simulink model "nomal_regulator"  (R2019a)
settings: Solver=FixedStepAuto  StartTime=0.0  StopTime=inf  FixedStep=sT  RelTol=1e-3  EnableMultiTasking=on
InitFcn:
  | clear;
  | init_robot;
  | param;
values from neighbouring files (symbols this model uses):
  g = 9.80665    [param.m]    (also in sim_param.m)
  inix = [0.00 0.00]'    [param.m]    (also in sim_param.m)
  iniXzmax = 0.05    [param.m]    (also in sim_param.m)
  iniXzmin = -0.05    [param.m]    (also in sim_param.m)
  iniy = [0.00 0.00]'    [param.m]    (also in sim_param.m)
  iniYzmax = 0.0625    [param.m]    (also in sim_param.m)
  iniYzmin = -0.0625    [param.m]    (also in sim_param.m)
  R = 20    [param.m]    (also in sim_param.m = 1)
  sT = 0.02    [param.m]    (also in sim_param.m = 0.001)
  w = sqrt(g/zc)    [param.m]    (also in sim_param.m)
undefined symbols (not defined in the file or in its folder): Ad, Bd, Cd, Dd, DiscIntNeverNeededParam, Discrete, fdesignblkfcn, gcbh, Time
libraries: raspberrypilib x6, cstblocks x5, dspfdesign x2, ctrlSharedLib x2
settings Model: SimulationMode=external  Creator=hideaki  LastModifiedBy=hideaki
settings SolverCC: PositivePriorityOrder=on
settings OptimizationCC: EnhancedBackFolding=on  PassReuseOutputArgsAs=Individual arguments  MaxStackSize=64  OptimizeBlockOrder=speed  DifferentSizesBufferReuse=on  OptimizationCustomize=off
settings DebuggingCC: ParameterTunabilityLossMsg=error  UnderSpecifiedDimensionMsg=warning
settings HardwareCC: ProdBitPerPointer=32  ProdBitPerSizeT=32  ProdBitPerPtrDiffT=32  ProdLargestAtomicInteger=Long  ProdLargestAtomicFloat=Double  ProdWordSize=32  ProdLongLongMode=on  ProdHWDeviceType=ARM Compatible->ARM Cortex  UseEmbeddedCoderFeatures=off  UseSimulinkCoderFeatures=off
settings SFSimCC: MATLABDynamicMemAlloc=off
settings RTWCC: SystemTargetFile=ert.tlc  HardwareBoard=Raspberry Pi  TLCOptions="-aInlineSetEventsForThisBaseRateFcn=TLC_FALSE -aSuppressMultiTaskScheduler=TLC_FALSE  -aRateBasedStepFcn=0"  TemplateMakefile=ert_default_tmf  RTWVerbose=off  Toolchain=GNU GCC Raspberry Pi  BuildConfiguration=Faster Runs  IncludeHyperlinkInReport=on
settings CodeAppCC: ForceParamTrailComments=on  OperatorAnnotations=on  SimulinkDataObjDesc=on  SFDataObjDesc=on  MangleLength=10  InsertBlockDesc=on
settings ERTTargetCC: SupportNonInlinedSFcns=on  SupportVariableSizeSignals=on  ExtMode=on  ExtModeMexArgs='192.168.10.103' 0 17725  ERTSrcFileBannerTemplate=codertarget_code_template.cgt  ERTHdrFileBannerTemplate=codertarget_code_template.cgt  ERTDataSrcFileTemplate=codertarget_code_template.cgt  ERTDataHdrFileTemplate=codertarget_code_template.cgt

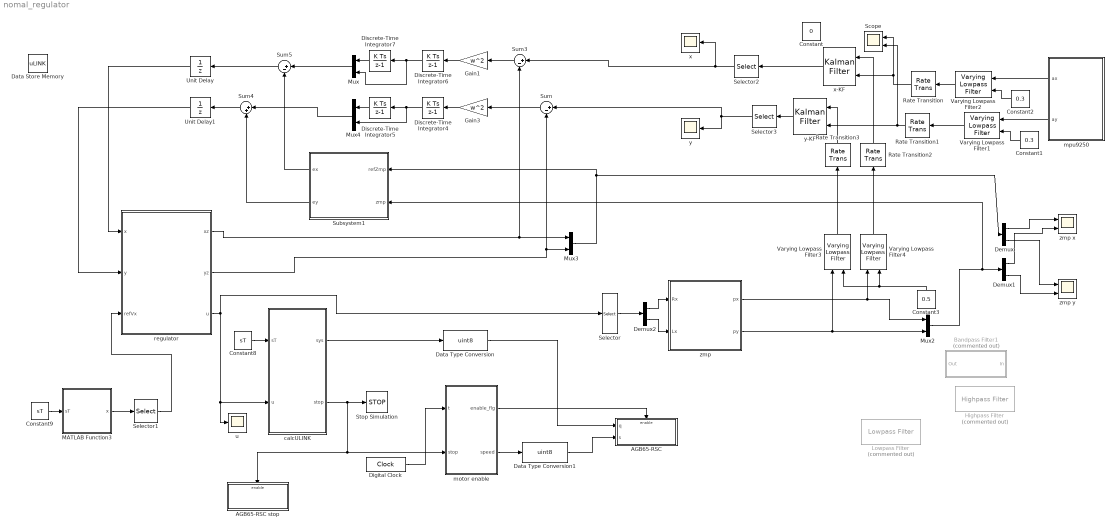
== system nomal_regulator ==
  AGB65-RSC : Subsystem  TreatAsAtomicUnit=on
  AGB65-RSC stop : Subsystem  TreatAsAtomicUnit=on
  Bandpass Filter1 : Subsystem  Commented=on  DialogController=fdesignblkfcn  InitFcn=fdesignblkfcn(gcbh, {'InitFcn'});  mask(Bandpass Filter){}
      mask help: Design a bandpass filter
      settings: CopyFcn=fdesignblkfcn(gcbh, {'CopyFcn'});
      mask Help: helpview(mapfilelocation('dsp'), 'dspbandpassfilter');
      mask Display: disp('Bandpass');
  Constant : Constant  Value=0
  Constant1 : Constant  Value=0.3
  Constant2 : Constant  Value=0.3
  Constant3 : Constant  Value=0.5
  Constant8 : Constant  Value=sT
  Constant9 : Constant  Value=sT
  Data Store Memory : DataStoreMemory  DataStoreName=uLINK  ReadBeforeWriteMsg=warning  WriteAfterWriteMsg=warning  WriteAfterReadMsg=warning  InitialValue=uLINK  ShowAdditionalParam=off  OutDataTypeStr=Bus: ULINK  Dimensions=[15 1]
  Data Type Conversion : DataTypeConversion  OutDataTypeStr=uint8
  Data Type Conversion1 : DataTypeConversion  OutDataTypeStr=uint8
  Demux : Demux  Outputs=2
  Demux1 : Demux  Outputs=2
  Demux2 : Demux  Outputs=2
  Digital Clock : DigitalClock  SampleTime=sT
  Discrete-Time Integrator{4..7} (4 alike) : DiscreteIntegrator  gainval=1  SampleTime=-1  ICPrevOutput=DiscIntNeverNeededParam  ICPrevScaledInput=DiscIntNeverNeededParam
  Gain1 : Gain  Gain=w^2
  Gain3 : Gain  Gain=w^2
  Highpass Filter : dspfdesign/Highpass Filter  Commented=on  FilterType=FIR  DesignForMinimumOrder=on  FilterOrder=50  StopbandFrequency=8e3  PassbandFrequency=12e3  StopbandAttenuation=80  PassbandRipple=0.1  InheritSampleRate=off  SampleRate=44100  SimulateUsing=Interpreted execution  roundingMode=Floor  coeffsDataTypeStr=fixdt(1,16)
      settings: SourceProductName=DSP System Toolbox
  Lowpass Filter : dspfdesign/Lowpass Filter  Commented=on  FilterType=FIR  DesignForMinimumOrder=on  FilterOrder=50  PassbandFrequency=8e3  StopbandFrequency=12e3  PassbandRipple=0.1  StopbandAttenuation=80  InheritSampleRate=off  SampleRate=44100  SimulateUsing=Interpreted execution  roundingMode=Floor  coeffsDataTypeStr=fixdt(1,16)
  MATLAB Function3 : MATLAB Function  TreatAsAtomicUnit=on  SystemSampleTime=sT
  Mux{,2..4} (4 alike) : Mux  Inputs=2
  Rate Transition{,1..3} (4 alike) : RateTransition
  Scope : Scope  NumInputPorts=2
  Selector : Selector  InputPortWidth=8  IndexOptions=Index vector (dialog)  Indices=[3 6]  OutputSizes=1
  Selector1 : Selector  InputPortWidth=3  IndexOptions=Index vector (dialog)  Indices=[2]  OutputSizes=1
  Selector2 : Selector  InputPortWidth=2  IndexOptions=Index vector (dialog)  Indices=[1]  OutputSizes=1
  Selector3 : Selector  InputPortWidth=2  IndexOptions=Index vector (dialog)  Indices=[1]  OutputSizes=1
  Stop Simulation : Stop
  Subsystem1 : Subsystem
  Sum : Sum  Inputs=|+-
  Sum3 : Sum  Inputs=|+-
  Sum4 : Sum  Inputs=|++
  Sum5 : Sum  Inputs=|+-
  Unit Delay : UnitDelay  SampleTime=-1  HasFrameUpgradeWarning=on
  Unit Delay1 : UnitDelay  SampleTime=-1  HasFrameUpgradeWarning=on
  Varying Lowpass Filter{1..4} (4 alike) : cstblocks/Linear Parameter Varying/Varying Lowpass Filter  N=1
      settings: SourceProductName=Control System Toolbox
  calcULINK : MATLAB Function  TreatAsAtomicUnit=on
  motor enable : MATLAB Function  TreatAsAtomicUnit=on
  mpu9250 : Subsystem
  regulator : Subsystem
  u : Scope
  x : Scope
  x-KF : ctrlSharedLib/Kalman Filter  TimeDomain=Discrete-Time  UseCurrentEstimator=on  ModelSource=Individual A, B, C, D matrices  ModelSourceVariable=ss(0.95,1,1,0,1)  A=Ad  B=Bd  C=Cd  D=Dd  NumberOfStates=1  NumberOfInputs=1  NumberOfOutputs=1  InitialEstimateSource=Dialog  X0=inix  P0=[100 50]'  UseK=off  UseGH=off  NumberOfProcessNoiseInputs=1  G=[0 0]'  TimeInvariantG=on  H=10  TimeInvariantH=on  Q=Q  TimeInvariantQ=on  R=R  TimeInvariantR=on  N=0  TimeInvariantN=on  AddInputPort=on  AddEnablePort=off  OutputEstimatedY=off  OutputP=off  Ts=sT
      settings: SourceProductBaseCode=CT
  y : Scope
  y-KF : ctrlSharedLib/Kalman Filter  TimeDomain=Discrete-Time  UseCurrentEstimator=on  ModelSource=Individual A, B, C, D matrices  ModelSourceVariable=ss(0.95,1,1,0,1)  A=Ad  B=Bd  C=Cd  D=Dd  NumberOfStates=1  NumberOfInputs=1  NumberOfOutputs=1  InitialEstimateSource=Dialog  X0=iniy  P0=10  UseK=off  UseGH=off  NumberOfProcessNoiseInputs=1  G=[0 0]'  TimeInvariantG=on  H=10  TimeInvariantH=on  Q=Q  TimeInvariantQ=on  R=R  TimeInvariantR=on  N=0  TimeInvariantN=on  AddInputPort=on  AddEnablePort=off  OutputEstimatedY=off  OutputP=off  Ts=sT
      settings: SourceProductBaseCode=CT
  zmp : Subsystem
  zmp x : Scope  NumInputPorts=2
  zmp y : Scope  NumInputPorts=2
  wires:
  Constant8/1 -> calcULINK/1(sT)
  Constant9/1 -> MATLAB Function3/1(sT)
  mpu9250/1(ax) -> Varying Lowpass Filter2/1
  Digital Clock/1 -> motor enable/1(t)
  Data Type Conversion1/1 -> AGB65-RSC/2(s)
  motor enable/1(enable_flg) -> AGB65-RSC/Enable
  Data Type Conversion/1 -> AGB65-RSC/1(q)
  calcULINK/1(sys) -> Data Type Conversion/1
  motor enable/2(speed) -> Data Type Conversion1/1
  calcULINK/2(stop) -> AGB65-RSC stop/Enable, motor enable/2(stop), Stop Simulation/1
  regulator/3(u) -> u/1, calcULINK/2(u), Selector/1
  Mux2/1 -> Subsystem1/2(zmp), Demux1/1
  Selector/1 -> Demux2/1
  Sum5/1 -> Unit Delay/1
  Sum4/1 -> Unit Delay1/1
  Mux3/1 -> Demux/1, Subsystem1/1(refZmp)
  MATLAB Function3/1(x) -> Selector1/1
  Selector1/1 -> regulator/3(refVx)
  zmp/1(px) -> Varying Lowpass Filter4/1, Mux2/1
  zmp/2(py) -> Mux2/2, Varying Lowpass Filter3/1
  Demux2/1 -> zmp/1(Rx)
  Demux2/2 -> zmp/2(Lx)
  Varying Lowpass Filter2/1 -> Rate Transition/1
  Selector2/1 -> x/1, Sum3/1
  regulator/1(xz) -> Mux3/1, Sum3/2
  regulator/2(yz) -> Mux3/2, Sum/2
  Mux/1 -> Sum5/1
  Demux/1 -> zmp x/1
  Demux1/1 -> zmp x/2
  Demux/2 -> zmp y/1
  Demux1/2 -> zmp y/2
  Discrete-Time Integrator5/1 -> Mux4/1
  Discrete-Time Integrator4/1 -> Discrete-Time Integrator5/1, Mux4/2
  Gain3/1 -> Discrete-Time Integrator4/1
  Sum/1 -> Gain3/1
  Mux4/1 -> Sum4/1
  Selector3/1 -> Sum/1, y/1
  mpu9250/2(ay) -> Varying Lowpass Filter1/1
  Varying Lowpass Filter1/1 -> Rate Transition1/1
  Sum3/1 -> Gain1/1
  Discrete-Time Integrator7/1 -> Mux/1
  Gain1/1 -> Discrete-Time Integrator6/1
  Discrete-Time Integrator6/1 -> Mux/2, Discrete-Time Integrator7/1
  x-KF/1 -> Selector2/1
  y-KF/1 -> Selector3/1
  Constant1/1 -> Varying Lowpass Filter1/2
  Rate Transition/1 -> Scope/1, x-KF/2
  Rate Transition1/1 -> Scope/2, y-KF/2
  Constant2/1 -> Varying Lowpass Filter2/2
  Unit Delay/1 -> regulator/1(x)
  Unit Delay1/1 -> regulator/2(y)
  Subsystem1/1(ex) -> Sum5/2
  Subsystem1/2(ey) -> Sum4/2
  Constant3/1 -> Varying Lowpass Filter3/2, Varying Lowpass Filter4/2
  Varying Lowpass Filter3/1 -> Rate Transition3/1
  Varying Lowpass Filter4/1 -> Rate Transition2/1
  Rate Transition2/1 -> x-KF/1
  Rate Transition3/1 -> y-KF/1

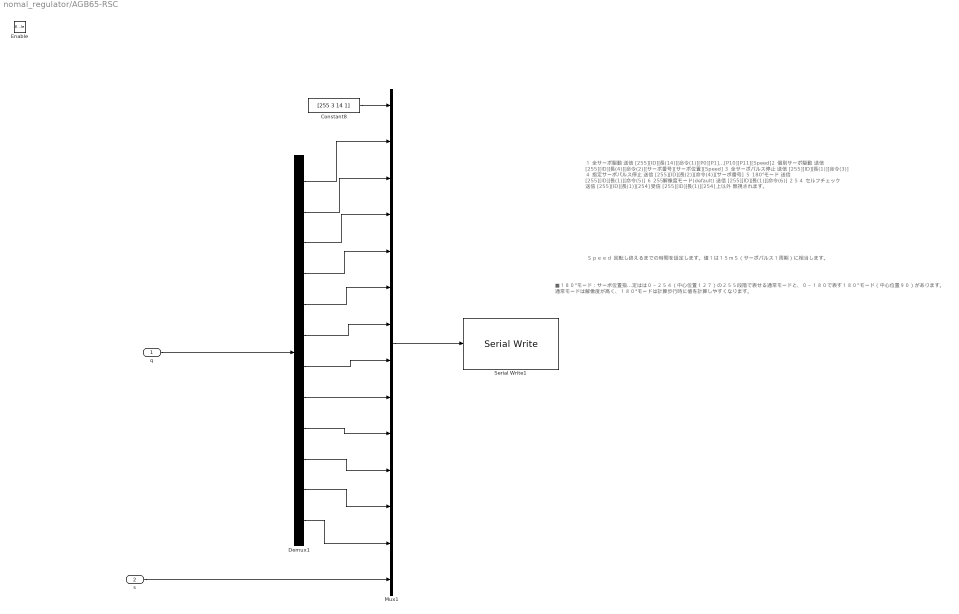
== system nomal_regulator/AGB65-RSC ==
  note: Ｓｐｅｅｄ 回転し終えるまでの時間を設定します。値１は１５ｍＳ（サーボパルス１周期）に相当します。
  note: １ 全サーボ駆動 送信 [255][ID][長(14)][命令(1)][P0][P1]...[P10][P11][Speed]
      | ２ 個別サーボ駆動 送信 [255][ID][長(4)][命令(2)][サーボ番号][サーボ位置][Speed]
      | ３ 全サーボパルス停止 送信 [255][ID][長(1)][命令(3)]
      | ４ 指定サーボパルス停止 送信 [255][ID][長(2)][命令(4)][サーボ番号]
      | ５ 180°モード 送信 [255][ID][長(1)][命令(5)]
      | ６ 255解像度モード(default) 送信 [255][ID][長(1)][命令(6)]
      | ２５４ セルフチェック 送信 [255][ID][長(1)][254] 受信 [255][ID][長(1)][254]
      | 上以外 無視されます。
  note: ■１８０°モード：サーボ位置指定はは０～２５４（中心位置１２７）の２５５段階で表せる通常モードと、０～１８０で表す１８０°モード（中心位置９０）があります。
      | 通常モードは解像度が高く、１８０°モードは計算歩行時に値を計算しやすくなります。
  q : Inport
  s : Inport  Port=2
  Enable : EnablePort
  Constant8 : Constant  Value=[255 3 14 1]  OutDataTypeStr=uint8
  Demux1 : Demux  Outputs=12
  Mux1 : Mux  Inputs=14
  Serial Write1 : raspberrypilib/Serial Write  Priority=1  board=Pi 3 Model B  SCIModule_=/dev/ttyS0  Baudrate_=115200  Parity=None  StopBits_=1  HardwareFlowControl=None  ByteOrder=LittleEndian  OutputStatus=off  blockPlatform=RaspberryPi
      settings: SourceProductName=Simulink Support Package for Raspberry Pi Hardware  SourceProductBaseCode=RASPPI
  wires:
  Constant8/1 -> Mux1/1
  Demux1/11 -> Mux1/12
  q/1 -> Demux1/1
  Demux1/1 -> Mux1/2
  Demux1/3 -> Mux1/4
  Demux1/2 -> Mux1/3
  Mux1/1 -> Serial Write1/1
  Demux1/6 -> Mux1/7
  Demux1/10 -> Mux1/11
  Demux1/5 -> Mux1/6
  Demux1/7 -> Mux1/8
  Demux1/8 -> Mux1/9
  s/1 -> Mux1/14
  Demux1/9 -> Mux1/10
  Demux1/12 -> Mux1/13
  Demux1/4 -> Mux1/5

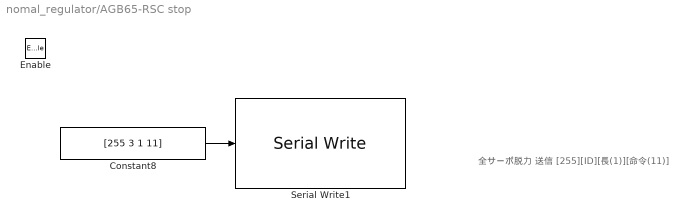
== system nomal_regulator/AGB65-RSC stop ==
  note: 全サーボ脱力 送信 [255][ID][長(1)][命令(11)]
  Enable : EnablePort
  Constant8 : Constant  Value=[255 3 1 11]  OutDataTypeStr=uint8
  Serial Write1 : raspberrypilib/Serial Write  Priority=1  board=Pi 3 Model B  SCIModule_=/dev/ttyS0  Baudrate_=115200  Parity=None  StopBits_=1  HardwareFlowControl=None  ByteOrder=LittleEndian  OutputStatus=off  blockPlatform=RaspberryPi
      settings: SourceProductName=Simulink Support Package for Raspberry Pi Hardware  SourceProductBaseCode=RASPPI
  wires:
  Constant8/1 -> Serial Write1/1

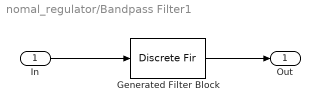
== system nomal_regulator/Bandpass Filter1 ==
  In : Inport
  Generated Filter Block : DiscreteFir  Tag=BlockMethodSubSystem  Coefficients=[-0.0118199987408042547 0.0121628797113327459 0.0187653420961211015 -0.0038859566916752521 0.00617302703660450782 -0.00799330781446441763 0.000649387236100319384 -0.00853505115886610786 -0.00350492002495765911 -0.00711106285974247646 -0.00734644359199590827 -0.00366446356246431793 -0.0101474907261420427 0.00166119112740601912 -0.0106818164382490588 0.00798118016776340478 -0.00794958057228637403 0.0136739609401164072 -0.0017104366339399206 0.0167318505505062096 0.00724764206845578129 0.0153031617213245236 0.0169724046181994881 0.00823820894327906283 0.0246104546693057119 -0.00429902872200196851 0.0270032365664331572 -0.0205818565716777424 0.0211767014494164546 -0.0374113276347360357 0.00493228214819367572 -0.0501802038611560974 -0.0229725070924577668 -0.0530003924446707797 -0.0641682213069025148 -0.0369265964862386248 -0.126487814949273442 0.0244803492939530132 -0.276321101997861363 0.548935421457220851 0.548935421457220851 -0.276321101997861363 0.0244803492939530132 -0.126487814949273442 -0.0369265964862386248 -0.0641682213069025148 -0.0530003924446707797 -0.0229725070924577668 -0.0501802038611560974 0.00493228214819367572 -0.0374113276347360357 0.0211767014494164546 -0.0205818565716777424 0.0270032365664331572 -0.00429902872200196851 0.0246104546693057119 0.00823820894327906283 0.0169724046181994881 0.0153031617213245236 0.00724764206845578129 0.0167318505505062096 -0.0017104366339399206 0.0136739609401164072 -0.00794958057228637403 0.00798118016776340478 -0.0106818164382490588 0.00166119112740601912 -0.0101474907261420427 -0.00366446356246431793 -0.00734644359199590827 -0.00711106285974247646 -0.00350492002495765911 -0.00853505115886610786 0.000649387236100319384 -0.00799330781446441763 0.00617302703660450782 -0.0038859566916752521 0.0187653420961211015 0.0121628797113327459 -0.0118199987408042547]  InputProcessing=Columns as channels (frame based)
  Out : Outport
  wires:
  In/1 -> Generated Filter Block/1
  Generated Filter Block/1 -> Out/1

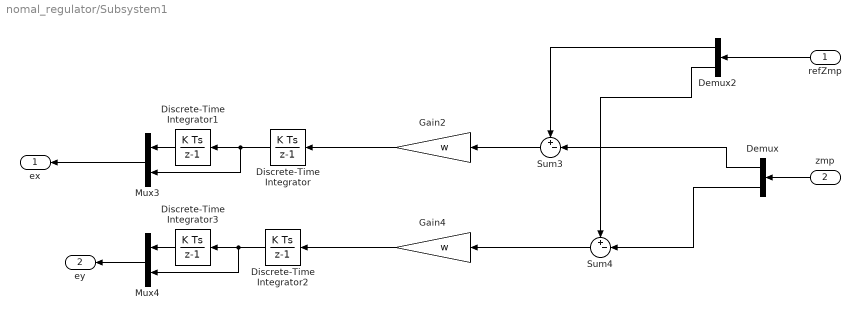
== system nomal_regulator/Subsystem1 ==
  refZmp : Inport
  zmp : Inport  Port=2
  Demux : Demux  Outputs=2
  Demux2 : Demux  Outputs=2
  Discrete-Time Integrator : DiscreteIntegrator  gainval=1  SampleTime=-1  ICPrevOutput=DiscIntNeverNeededParam  ICPrevScaledInput=DiscIntNeverNeededParam
  Discrete-Time Integrator1 : DiscreteIntegrator  SampleTime=-1  ICPrevOutput=DiscIntNeverNeededParam  ICPrevScaledInput=DiscIntNeverNeededParam
  Discrete-Time Integrator2 : DiscreteIntegrator  gainval=1  SampleTime=-1  ICPrevOutput=DiscIntNeverNeededParam  ICPrevScaledInput=DiscIntNeverNeededParam
  Discrete-Time Integrator3 : DiscreteIntegrator  SampleTime=-1  ICPrevOutput=DiscIntNeverNeededParam  ICPrevScaledInput=DiscIntNeverNeededParam
  Gain2 : Gain  Gain=w
  Gain4 : Gain  Gain=w
  Mux3 : Mux  Inputs=2
  Mux4 : Mux  Inputs=2
  Sum3 : Sum  Inputs=+-|
  Sum4 : Sum  Inputs=+-|
  ex : Outport
  ey : Outport  Port=2
  wires:
  Demux2/1 -> Sum3/1
  Discrete-Time Integrator2/1 -> Discrete-Time Integrator3/1, Mux4/2
  Demux/1 -> Sum3/2
  Discrete-Time Integrator3/1 -> Mux4/1
  Mux3/1 -> ex/1
  Discrete-Time Integrator1/1 -> Mux3/1
  Demux2/2 -> Sum4/1
  Discrete-Time Integrator/1 -> Mux3/2, Discrete-Time Integrator1/1
  Mux4/1 -> ey/1
  Demux/2 -> Sum4/2
  Sum3/1 -> Gain2/1
  zmp/1 -> Demux/1
  Sum4/1 -> Gain4/1
  refZmp/1 -> Demux2/1
  Gain4/1 -> Discrete-Time Integrator2/1
  Gain2/1 -> Discrete-Time Integrator/1

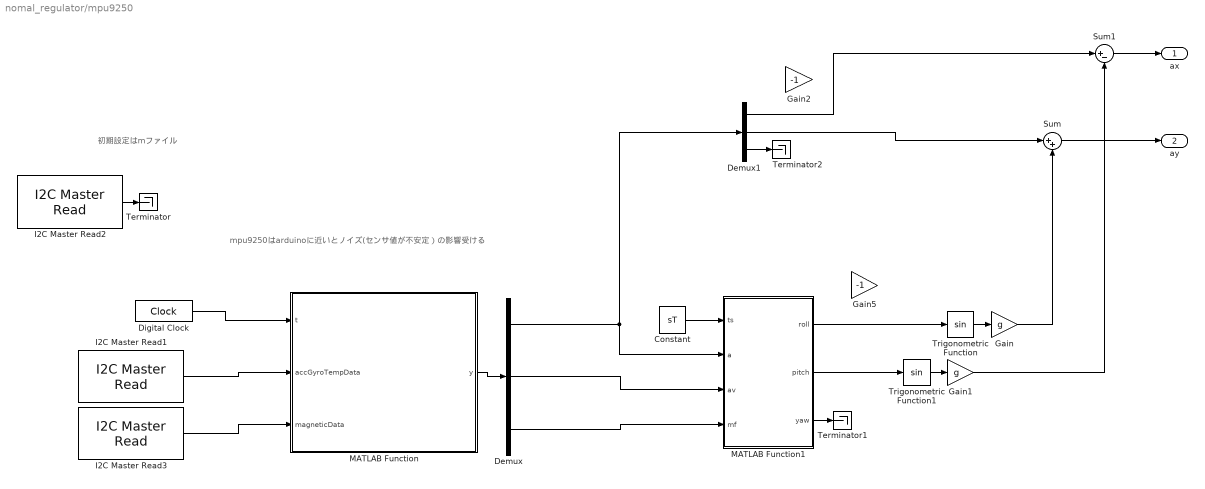
== system nomal_regulator/mpu9250 ==
  note: mpu9250はarduinoに近いとノイズ(センサ値が不安定）の影響受ける
  note: 初期設定はmファイル
  Constant : Constant  Value=sT
  Demux : Demux  Outputs=3
  Demux1 : Demux  Outputs=3
  Digital Clock : DigitalClock  SampleTime=sT
  Gain : Gain  Gain=g
  Gain1 : Gain  Gain=g
  Gain2 : Gain  Gain=-1
  Gain5 : Gain  Gain=-1
  I2C Master Read1 : raspberrypilib/I2C Master Read  BoardProperty=Pi 3 Model B  Mode=Master  SlaveAddress=hex2dec( '68' )  SlaveByteOrder=BigEndian  Direction=Receiver  RegisterAddressMode=on  RegisterAddress=hex2dec( '3b' )  SlaveDataType=uint8  DataLength=14  NoAck=off  RepeatedStart=off  OutputStatus=off  SampleTime=-1
      settings: SourceProductName=Simulink Support Package for Raspberry Pi Hardware  SourceProductBaseCode=RASPPI
  I2C Master Read2 : raspberrypilib/I2C Master Read  BoardProperty=Pi 3 Model B  Mode=Master  SlaveAddress=hex2dec( '0c' )  SlaveByteOrder=BigEndian  Direction=Receiver  RegisterAddressMode=on  RegisterAddress=hex2dec( '02' )  SlaveDataType=uint8  DataLength=1  NoAck=off  RepeatedStart=off  OutputStatus=off  SampleTime=-1
      settings: SourceProductName=Simulink Support Package for Raspberry Pi Hardware  SourceProductBaseCode=RASPPI
  I2C Master Read3 : raspberrypilib/I2C Master Read  BoardProperty=Pi 3 Model B  Mode=Master  SlaveAddress=hex2dec( '0c' )  SlaveByteOrder=BigEndian  Direction=Receiver  RegisterAddressMode=on  RegisterAddress=hex2dec( '03' )  SlaveDataType=uint8  DataLength=7  NoAck=off  RepeatedStart=off  OutputStatus=off  SampleTime=-1
      settings: SourceProductName=Simulink Support Package for Raspberry Pi Hardware  SourceProductBaseCode=RASPPI
  MATLAB Function : MATLAB Function  TreatAsAtomicUnit=on
  MATLAB Function1 : MATLAB Function  TreatAsAtomicUnit=on
  Sum : Sum  Inputs=|++
  Sum1 : Sum  Inputs=|+-
  Terminator : Terminator
  Terminator1 : Terminator
  Terminator2 : Terminator
  Trigonometric Function : Trigonometry
  Trigonometric Function1 : Trigonometry
  ax : Outport
  ay : Outport  Port=2
  wires:
  I2C Master Read2/1 -> Terminator/1
  Constant/1 -> MATLAB Function1/1(ts)
  I2C Master Read3/1 -> MATLAB Function/3(magneticData)
  Demux/2 -> MATLAB Function1/3(av)
  Sum/1 -> ay/1
  Demux/1 -> Demux1/1, MATLAB Function1/2(a)
  Demux/3 -> MATLAB Function1/4(mf)
  Gain/1 -> Sum/2
  I2C Master Read1/1 -> MATLAB Function/2(accGyroTempData)
  Trigonometric Function/1 -> Gain/1
  Sum1/1 -> ax/1
  Trigonometric Function1/1 -> Gain1/1
  MATLAB Function1/2(pitch) -> Trigonometric Function1/1
  Gain1/1 -> Sum1/2
  MATLAB Function1/1(roll) -> Trigonometric Function/1
  Demux1/1 -> Sum1/1
  Digital Clock/1 -> MATLAB Function/1(t)
  MATLAB Function/1(y) -> Demux/1
  MATLAB Function1/3(yaw) -> Terminator1/1
  Demux1/3 -> Terminator2/1
  Demux1/2 -> Sum/1

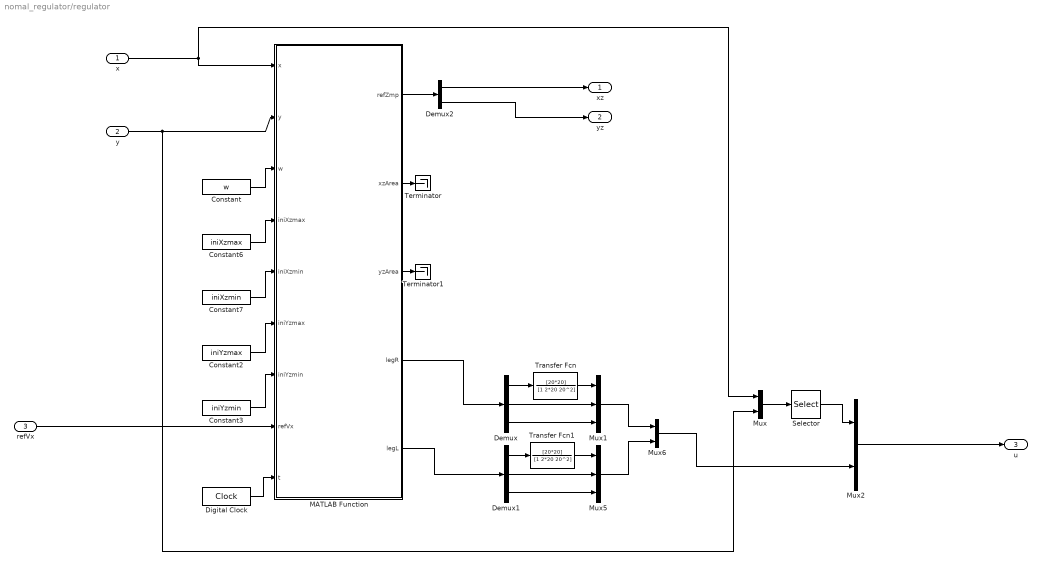
== system nomal_regulator/regulator ==
  x : Inport
  y : Inport  Port=2
  refVx : Inport  Port=3
  Constant : Constant  Value=w
  Constant2 : Constant  Value=iniYzmax
  Constant3 : Constant  Value=iniYzmin
  Constant6 : Constant  Value=iniXzmax
  Constant7 : Constant  Value=iniXzmin
  Demux : Demux  Outputs=3
  Demux1 : Demux  Outputs=3
  Demux2 : Demux  Outputs=2
  Digital Clock : DigitalClock  SampleTime=sT
  MATLAB Function : MATLAB Function  TreatAsAtomicUnit=on  SystemSampleTime=sT
  Mux : Mux  Inputs=2
  Mux1 : Mux  Inputs=3
  Mux2 : Mux  Inputs=2
  Mux5 : Mux  Inputs=3
  Mux6 : Mux  Inputs=2
  Selector : Selector  InputPortWidth=4  IndexOptions=Index vector (dialog)  Indices=[1 3]  OutputSizes=1
  Terminator : Terminator
  Terminator1 : Terminator
  Transfer Fcn : TransferFcn  Numerator=[20*20]  Denominator=[1 2*20 20^2]
  Transfer Fcn1 : TransferFcn  Numerator=[20*20]  Denominator=[1 2*20 20^2]
  xz : Outport
  yz : Outport  Port=2
  u : Outport  Port=3
  wires:
  Constant/1 -> MATLAB Function/3(w)
  MATLAB Function/4(legR) -> Demux/1
  Transfer Fcn1/1 -> Mux5/1
  Constant3/1 -> MATLAB Function/7(iniYzmin)
  Mux2/1 -> u/1
  MATLAB Function/1(refZmp) -> Demux2/1
  Constant2/1 -> MATLAB Function/6(iniYzmax)
  Transfer Fcn/1 -> Mux1/1
  x/1 -> MATLAB Function/1(x), Mux/1
  Demux/3 -> Mux1/3
  Demux2/1 -> xz/1
  MATLAB Function/5(legL) -> Demux1/1
  Demux1/2 -> Mux5/2
  Demux/1 -> Transfer Fcn/1
  Demux1/3 -> Mux5/3
  Selector/1 -> Mux2/1
  Mux/1 -> Selector/1
  Demux2/2 -> yz/1
  Constant7/1 -> MATLAB Function/5(iniXzmin)
  Demux1/1 -> Transfer Fcn1/1
  Mux5/1 -> Mux6/2
  Constant6/1 -> MATLAB Function/4(iniXzmax)
  Mux6/1 -> Mux2/2
  Demux/2 -> Mux1/2
  Mux1/1 -> Mux6/1
  Digital Clock/1 -> MATLAB Function/9(t)
  refVx/1 -> MATLAB Function/8(refVx)
  MATLAB Function/2(xzArea) -> Terminator/1
  MATLAB Function/3(yzArea) -> Terminator1/1
  y/1 -> Mux/2, MATLAB Function/2(y)

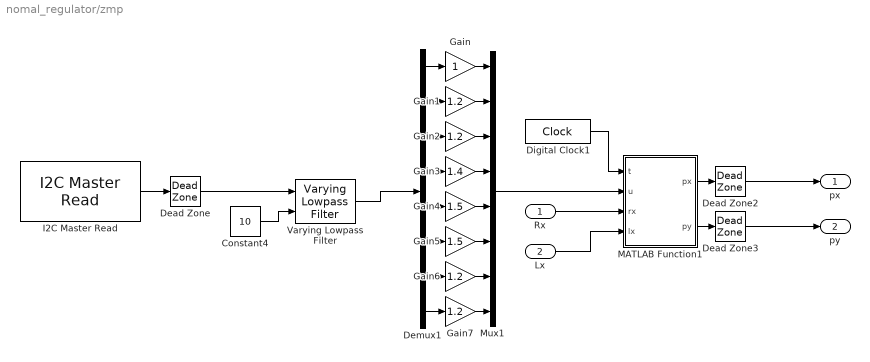
== system nomal_regulator/zmp ==
  Rx : Inport
  Lx : Inport  Port=2
  Constant4 : Constant  Value=10
  Dead Zone : DeadZone  LowerValue=0  UpperValue=5  SaturateOnIntegerOverflow=on
  Dead Zone2 : DeadZone  LowerValue=-1e-5  UpperValue=1e-5  SaturateOnIntegerOverflow=on
  Dead Zone3 : DeadZone  LowerValue=-1e-5  UpperValue=1e-5  SaturateOnIntegerOverflow=on
  Demux1 : Demux  Outputs=8
  Digital Clock1 : DigitalClock  SampleTime=sT
  Gain : Gain
  Gain{1..2,6..7} (4 alike) : Gain  Gain=1.2
  Gain3 : Gain  Gain=1.4
  Gain4 : Gain  Gain=1.5
  Gain5 : Gain  Gain=1.5
  I2C Master Read : raspberrypilib/I2C Master Read  BoardProperty=Pi 3 Model B  Mode=Master  SlaveAddress=hex2dec( '04' )  SlaveByteOrder=BigEndian  Direction=Receiver  RegisterAddressMode=off  RegisterAddress=hex2dec( '20' )  SlaveDataType=uint8  DataLength=8  NoAck=off  RepeatedStart=off  OutputStatus=off  SampleTime=sT
      settings: SourceProductName=Simulink Support Package for Raspberry Pi Hardware  SourceProductBaseCode=RASPPI
  MATLAB Function1 : MATLAB Function  TreatAsAtomicUnit=on
  Mux1 : Mux  Inputs=8
  Varying Lowpass Filter : cstblocks/Linear Parameter Varying/Varying Lowpass Filter  N=1
      settings: SourceProductName=Control System Toolbox
  px : Outport
  py : Outport  Port=2
  wires:
  Mux1/1 -> MATLAB Function1/2(u)
  Demux1/5 -> Gain4/1
  Demux1/6 -> Gain5/1
  Varying Lowpass Filter/1 -> Demux1/1
  Constant4/1 -> Varying Lowpass Filter/2
  I2C Master Read/1 -> Dead Zone/1
  Demux1/1 -> Gain/1
  Gain/1 -> Mux1/1
  Gain2/1 -> Mux1/3
  Gain4/1 -> Mux1/5
  Gain1/1 -> Mux1/2
  MATLAB Function1/1(px) -> Dead Zone2/1
  Gain3/1 -> Mux1/4
  Gain6/1 -> Mux1/7
  Gain7/1 -> Mux1/8
  Dead Zone/1 -> Varying Lowpass Filter/1
  Demux1/3 -> Gain2/1
  Demux1/7 -> Gain6/1
  Demux1/2 -> Gain1/1
  Digital Clock1/1 -> MATLAB Function1/1(t)
  Demux1/8 -> Gain7/1
  Gain5/1 -> Mux1/6
  Demux1/4 -> Gain3/1
  MATLAB Function1/2(py) -> Dead Zone3/1
  Dead Zone2/1 -> px/1
  Rx/1 -> MATLAB Function1/3(rx)
  Lx/1 -> MATLAB Function1/4(lx)
  Dead Zone3/1 -> py/1

== matlab function nomal_regulator/motor enable ==
  data: t input; enable_flg output; speed output; stop input
function [enable_flg,speed]= fcn(t,stop)
    
    enable_flg = 0;
    speed = 1;
    persistent cnt;
    if isempty(cnt)
        cnt = 0;
    end
    
    if (stop == 1) 
        enable_flg = 0;
    else
        if (cnt == 0)
            enable_flg = 1;
            speed = 30;
            cnt = cnt+1;
        elseif (t <= 5)
            enable_flg = 0;
        else
            enable_flg = 1;
        end
    end
end

== matlab function nomal_regulator/regulator/MATLAB Function ==
  data: refZmp output size=2; xzArea output size=2; yzArea output size=2; x input; legR output size=3; legL output size=3; y input; w input; iniXzmax input; iniXzmin input; iniYzmax input; iniYzmin input; refVx input; t input
function [refZmp,xzArea,yzArea,legR,legL] = fcn(x,y,w,iniXzmax,iniXzmin,iniYzmax,iniYzmin,refVx,t)
    
    
    %% x軸
    qx = 0.5;
    persistent xR;
    if isempty(xR)
        xR = 0.0;
    end
    persistent xL;
    if isempty(xL)
        xL = 0.0;
    end
    
    %% y軸
    qy = 0.5;
    %r 振幅
    r = 0.03;
    k = 1;
    persistent rho;
    if isempty(rho)
        rho = 1;
    end
    
    %% z軸
    %左足裏内側縁
    xLin = 0.0175;
    %右足裏内側縁
    xRin = -0.0175;
    
    %% y軸
    refy = 0.0;
    zeta = sqrt( (y(1)-refy)^2 + (y(2)^2/(w^2*qy)) );
    f = 1-rho*exp( k*(1-((qy+1)^2*zeta^2)/r^2) );
    yz = refy+(qy+1)*(y(1)-refy + f*(y(2)/w));
    
    yzmax = iniYzmax;
    yzmin = iniYzmin;
    Yz = yz -refy;
    
    %% z軸   
    %右足高さ
    zR = clac(Yz,y,w,rho,xLin,r);
    if (zR > 0) 
        yzmin = refy + xLin;
    end
    %左足高さ
    zL = clac(Yz,y,w,rho,xRin,r);
    if (zL > 0) 
        yzmax = refy + xRin;
    end
    
    if (yz > yzmax)
        yz = yzmax;
    elseif (yz < yzmin)
        yz = yzmin;
    end
    
    refys = y(1)+(y(2)/w);
    yR = -0.04;
    yL = 0.04;
    
    %% x軸
    
    xzmax = iniXzmax;
    xzmin = iniXzmin;
        
    refx = x(1);
    if (refVx == 0) 
        %立位可安定
        qx = 1.0;
    else
        %速度追従
        qx = 0.0;
    end
    
    %ZMP
    xz = refx+(qx+1)*(x(1)-refx + (x(2)-refVx)/w);
    %着地位置
    refxs = x(1)+(x(2)/w);
    
    if (zR > 0)
        xR = refxs;
        xzmax = xL + iniXzmax;
        xzmin = xL + iniXzmin;
    elseif (zL > 0)
        xL = refxs;
        xzmax = xR + iniXzmax;
        xzmin = xR + iniXzmin;
    else
        if (xL > xR)
            xzmax = xL + iniXzmax;
            xzmin = xR + iniXzmin;
        else
            xzmax = xR + iniXzmax;
            xzmin = xL + iniXzmin;
        end
    end
    
    if (xz > xzmax)
        xz = xzmax;
    elseif (xz < xzmin)
        xz = xzmin;
    end
    
    refZmp = zeros(2,1);    
    legR = [0 yR 0]';
    legL = [0 yL 0]';
    
    xzArea = [xzmax xzmin]';
    yzArea = [yzmax yzmin]';
    
    if (t >= 5)
        refZmp = [xz yz]';
        legR = [xR yR zR]';
        legL = [xL yL zL]';
    end
    
end

%% 
function z = clac(yz,x,w,rho,xLin,r)
    
    q = 0.5;
    h = 0.012;
     
    pz = yz - ((q+1)*x(2)/w*sqrt(q))*1i;
    
    %軸足内側に入った
    pLin = xLin - sqrt(complex(abs(pz)^2-xLin^2))*1i;
    %軸足内側から出た
    pLout = xLin + sqrt(complex(abs(pz)^2-xLin^2))*1i;
    
    z = 0;
    phiL = 0;
    %左が軸足
    if (xLin > 0)
        %ZMPが左足にある
        if (real(pz) > xLin)
            %plinからpzまでの角度
            ang_pz = angle(pz)-angle(pLin);
            %pLinからpLoutまでの角度
            ang_io = angle(pLout)-angle(pLin);
            phiL = ang_pz/ang_io;
        end
    %右が軸足
    else
        %ZMPが右足にある
        if (real(pz) < xLin)
            %plinからpzまでの角度（負なので正（第一、第二象限）に移す）
            ang_pz = 0;
            if (angle(pz) > 0) 
                ang_pz = angle(pz)-pi+angle(pLin)+pi; 
            else
                ang_pz = angle(pz)+pi+angle(pLin)+pi; 
            end
            %pLinからpLoutまでの角度（負なので正（第一、第二象限）に移す）
            ang_io = angle(pLin)+pi-angle(pLout)+pi;
            phiL = ang_pz/ang_io;
        end
    end
    
    if (0 < phiL && phiL < 1)
        z = (1/2)*(h*abs(pz)/r)*sigma(rho)*(1-cos(2*pi*phiL));
    end
end

function y = sigma(rho)
    
    if (rho > 1)
        y = 1;
    elseif (exp(-1) <= rho && rho <= 1)
        y = (rho-exp(-1))/(1-exp(-1));
    else
        y = 0;
    end
end

== matlab function nomal_regulator/mpu9250/MATLAB Function ==
  settings: updateMethod=DISCRETE
  data: t input; accGyroTempData input; y output; magneticData input
function y = out_mpu9250(t,accGyroTempData,magneticData)

    y = zeros(9,1);
    
    %計算で使用するので，選択したレンジを入力する
    accRange = 16.0;
    %%計算で使用するので，選択したレンジを入力する
    gyroRange = 2000.0;
    
    %%Acc
    ax = -nbin2dec(dec2bin(bitshift(uint16(accGyroTempData(1)),8) + uint16(accGyroTempData(2)),16));
    ay = nbin2dec(dec2bin(bitshift(uint16(accGyroTempData(3)),8) + uint16(accGyroTempData(4)),16));
    az = nbin2dec(dec2bin(bitshift(uint16(accGyroTempData(5)),8) + uint16(accGyroTempData(6)),16));
    
    %%Gyro
    gx = nbin2dec(dec2bin(bitshift(uint16(accGyroTempData(9)),8) + uint16(accGyroTempData(10)),16));
    gy = nbin2dec(dec2bin(bitshift(uint16(accGyroTempData(11)),8) + uint16(accGyroTempData(12)),16));
    gz = nbin2dec(dec2bin(bitshift(uint16(accGyroTempData(13)),8) + uint16(accGyroTempData(14)),16));
    
    %%Temp
    %tempMPU9250Raw = bitshift(accGyroTempData(7),8) | accGyroTempData(8);%accGyroTempData[6]を左に8シフトし(<<)，accGyroTempData[7]を足し合わせる(|)
    
    %%Magneto
    mx = nbin2dec(dec2bin(bitshift(uint16(magneticData(4)),8) + uint16(magneticData(3)),16));
    my = nbin2dec(dec2bin(bitshift(uint16(magneticData(2)),8) + uint16(magneticData(1)),16));
    mz = -(nbin2dec(dec2bin(bitshift(uint16(magneticData(6)),8) + uint16(magneticData(5)),16)));
    
    %加速度
    %16bit(最大値32768)を16Gで割る
    ax = ax * accRange / 32768.0;%[G]に変換
    ay = ay * accRange / 32768.0;%[G]に変換
    az = az * accRange / 32768.0;%[G]に変換
    
    %角加速度
    gx = gx * gyroRange / 32768.0;%[deg/s]に変換
    gy = gy * gyroRange / 32768.0;%[deg/s]に変換
    gz = gz * gyroRange / 32768.0;%[deg/s]に変換
    
    persistent idx; 
    if isempty(idx) 
        idx = 1; 
    end
    
    %最初の100までの平均値
    persistent ax_100;
    persistent ay_100;
    %persistent az_100;
    persistent ax_avg;
    persistent ay_avg;
    %persistent az_avg;
    
    persistent gx_100;
    persistent gy_100;
    persistent gz_100;
    persistent gx_avg;
    persistent gy_avg;
    persistent gz_avg;
    if isempty(gx_100)
        ax_100 = zeros(1, 100);
        ay_100 = zeros(1, 100);
        %az_100 = zeros(1, 100);
        ax_avg = 0;
        ay_avg = 0;
        %az_avg = 0;
        
        gx_100 = zeros(1, 100);
        gy_100 = zeros(1, 100);
        gz_100 = zeros(1, 100);
        gx_avg = 0;
        gy_avg = 0;
        gz_avg = 0;
    end
    
    y = zeros(9,1);
    if (t < 2)
        
    elseif (t >= 2 && idx <= 100)
        ax_100(idx) = ax;
        ay_100(idx) = ay;
        %az_100(idx) = az;
        ax_avg = mean(ax_100);
        ay_avg = mean(ay_100);
        %az_avg = mean(az_100);
        
        gx_100(idx) = gx;
        gy_100(idx) = gy;
        gz_100(idx) = gz;
        gx_avg = mean(gx_100);
        gy_avg = mean(gy_100);
        gz_avg = mean(gz_100);
        
        idx = idx+1;
        
    else
        
        ax = ax-ax_avg;
        ay = ay-ay_avg;
        %az = az-az_avg;
        
        gx = gx-gx_avg;
        gy = gy-gy_avg;
        gz = gz-gz_avg;
        
        %[G]→[m/s^2]
        y(1) = ax*9.80665;
        y(2) = ay*9.80665;
        y(3) = az*9.80665;

        y(4) = deg2rad(gx);
        y(5) = deg2rad(gy);
        y(6) = deg2rad(gz);

        %tempMPU9250 = ((tempMPU9250Raw - 0.0) / 333.87) + 21.0;

        %方位
        mx = mx / 32768.0 * 4800.0;%[uT]に変換
        my = my / 32768.0 * 4800.0;%[uT]に変換
        mz = mz / 32768.0 * 4800.0;%[uT]に変換

        %感度とオフセット
        Gx = 1;
        bx = 27.4;
        Gy = 0.9;
        by = 9;
        Gz = 1;
        bz = 30;

        %パラメータ補正
        mfx = (mx-bx)/Gx;
        mfy = (my-by)/Gy;
        mfz = (mz-bz)/Gz;

        y(7) = mfx;
        y(8) = mfy;
        y(9) = mfz;
    end
    
    
end

== matlab function nomal_regulator/mpu9250/MATLAB Function1 ==
  settings: updateMethod=DISCRETE
  data: ts input; a input; av input; roll output; mf input; pitch output; yaw output
function [roll, pitch, yaw] = kf(ts, a, av, mf)
    
    persistent cnt;
    if isempty(cnt)
        cnt = 0;
    end
    if (cnt < 102)
        cnt = cnt+1;
    end
    
    persistent x;
    if isempty(x)
        x = zeros(3, 1);
    end
    persistent P;
    if isempty(P)
        P = 0.1*eye(3);
    end
    
    persistent yawm_100;
    persistent yawm_avg;
    if isempty(yawm_100)
        yawm_100 = zeros(1, 100);
        yawm_avg = 0;
    end
    
    roll = 0;
    pitch = 0;
    yaw = 0;
        
    rolla = atan2(a(2), a(3));
    pitcha = atan2(-a(1), sqrt(a(2)*a(2)+a(3)*a(3)));
    
    if (cnt <= 100)
        
        %傾斜誤差補正
        M = [cos(pitcha) sin(rolla)*sin(pitcha) cos(rolla)*sin(pitcha);
            0 cos(rolla) -sin(rolla);
            -sin(pitcha) sin(rolla)*cos(pitcha) cos(rolla)*cos(pitcha)];
        m = M*[mf(1);mf(2);mf(3)];

        %yaw
        yawm = atan2(-m(2), m(1));
        yawm_100(cnt) = yawm;
        yawm_avg = mean(yawm_100(cnt));
        
        x(1) = yawm;
        x(2) = pitcha;
        x(3) = rolla;
        
        roll = rolla;
        pitch = pitcha;
        yaw = yawm-yawm_avg;
        %yaw = yawm;
        
    else
        
        I = eye(3);
        
        %%共分散行列
        Q = [160 0 0;
            0 160 0;
            0 0 160];
        R = [20 0 0;
            0 20 0;
            0 0 20];
        
        B = [0 sin(x(3))/cos(x(2)) cos(x(3))/cos(x(2));
            0 cos(x(3)) -sin(x(3));
            1 sin(x(3))*tan(x(2)) cos(x(3))*tan(x(2))];
        
        u = [av(1)*ts;av(2)*ts;av(3)*ts];
        
        %%傾斜誤差補正
        M = [cos(x(2)) sin(x(3))*sin(x(2)) cos(x(3))*sin(x(2));
            0 cos(x(3)) -sin(x(3));
            -sin(x(2)) sin(x(3))*cos(x(2)) cos(x(3))*cos(x(2))];
        m = M*[mf(1);mf(2);mf(3)];

        yawm = atan2(-m(2), m(1))-yawm_avg;
        %yawm = atan2(-m(2), m(1));
        
        y = [yawm;pitcha;rolla];
        
        %%カルマンフィルタ
        x = I*x+B*u;
        P = I*P*I'+Q;
        K = (P*I')/(I*P*I'+R);
        x = x+K*(y-I*x);
        P = (I-K*I)*P;
        
        roll = x(3);
        pitch = x(2);
        yaw = x(1);
        
    end
    
end

== matlab function nomal_regulator/calcULINK ==
  settings: updateMethod=DISCRETE
  data: sT input; u input; sys output; uLINK data_store_memory; stop output
function [sys,stop] = calcULINK(sT,u)

    %u[腰X 腰Y 右足X 右足Y 右足Z 左足X 左足Y 左足Z]
    
    stop = 0;
    global uLINK;
    
    persistent cnt;
    if isempty(cnt)
        cnt = 0.0;
    end
    
    ToDeg = 180/pi;
    ToRad = pi/180;
    
    sys = zeros(12,1);
    
    %%% ZMPの計算
    %com = calcCoM;  % 重心位置
    %P = calcP(1);   % 並進運動量
    %L = calcL(1);   % 原点回りの角運動量
    
    %Zc  = com(3);      % 線形倒立振子の設定高さ
    %Tc  = sqrt(Zc/G);  % 線形倒立振子の時定数
    %cx0 = com(1);
    %cy0 = com(2);
    
    
    p0 = uLINK(JointName.BODY).p;
    uLINK(JointName.BODY).p = [u(1), u(2), uLINK(JointName.BODY).p(3)]';
    v = (uLINK(JointName.BODY).p-p0)/sT;
    uLINK(JointName.BODY).v = [v(1) v(2) v(3)]';
    uLINK(JointName.BODY).R = RPY2R([0 0*ToRad 0]);

    %ForwardKinematics(1);
    
    p = [u(3) u(4) u(5)]';
    Rfoot.p = [u(3) u(4) u(5)]';
    Rfoot.R = RPY2R([0 0 0]);
    v = (p-uLINK(JointName.RLEG_FOOT).p)/sT;
    Rfoot.v = [v(1) v(2) v(3)]';
    Rfoot.w = [0 0 0]';
    InverseKinematicsAll(8, Rfoot);
    
    p = [u(6) u(7) u(8)]';
    Lfoot.p = [u(6) u(7) u(8)]';
    Lfoot.R = RPY2R([0 0 0]);
    v = (p-uLINK(JointName.LLEG_FOOT).p)/sT;
    Lfoot.v = [v(1) v(2) v(3)]';
    Lfoot.w = [0 0 0]';
    InverseKinematicsAll(15, Lfoot);
    
    ForwardVelocity(1); 
    
    
    
    sys = [90 90 90 90 90 90 90 90 90 90 90 90]';
    
    if (abs(rad2deg(uLINK(JointName.RLEG_J0).q)) > 30 || abs(rad2deg(uLINK(JointName.LLEG_J0).q)) > 30)
        stop = 1;
    end
    if (abs(rad2deg(uLINK(JointName.RLEG_J1).q)) > 60 || abs(rad2deg(uLINK(JointName.LLEG_J1).q)) > 60 || ...
        abs(rad2deg(uLINK(JointName.RLEG_J5).q)) > 60 || abs(rad2deg(uLINK(JointName.LLEG_J5).q)) > 60)
        stop = 1;
    end
    if (abs(rad2deg(uLINK(JointName.RLEG_J2).q)) > 60 || abs(rad2deg(uLINK(JointName.LLEG_J2).q)) > 60 || ...
        abs(rad2deg(uLINK(JointName.RLEG_J4).q)) > 60 || abs(rad2deg(uLINK(JointName.LLEG_J4).q)) > 60)
        stop = 1;
    end
    if (abs(rad2deg(uLINK(JointName.RLEG_J3).q)) > 90 || abs(rad2deg(uLINK(JointName.LLEG_J3).q)) > 90)
        stop = 1;
    end
    
    sys(1) = round(rad2deg(uLINK(JointName.RLEG_J0).q))+90;
    %股関節の剛性不足による胴体の傾き補償フィードフォワード
    sys(2) = round(rad2deg(uLINK(JointName.RLEG_J1).q))+90-1;
    sys(3) = -round(rad2deg(uLINK(JointName.RLEG_J2).q))+90;
    sys(4) = -round(rad2deg(uLINK(JointName.RLEG_J3).q))+90;
    sys(5) = -round(rad2deg(uLINK(JointName.RLEG_J4).q))+90;
    sys(6) = -round(rad2deg(uLINK(JointName.RLEG_J5).q))+90;
    
    sys(7) = round(rad2deg(uLINK(JointName.LLEG_J0).q))+90;
    sys(8) = round(rad2deg(uLINK(JointName.LLEG_J1).q))+90+1;
    sys(9) = -round(rad2deg(uLINK(JointName.LLEG_J2).q))+90;
    sys(10) = -round(rad2deg(uLINK(JointName.LLEG_J3).q))+90;
    sys(11) = -round(rad2deg(uLINK(JointName.LLEG_J4).q))+90;
    sys(12) = -round(rad2deg(uLINK(JointName.LLEG_J5).q))+90;
    
    for i = 1:12
        if (abs(sys(i)) > 180)
            stop = 1;
        end
    end
   
    
    cnt = cnt + sT;
end

== matlab function nomal_regulator/MATLAB Function3 ==
  data: x output; sT input
function x = orbit(sT)

    persistent t; 
    if (isempty(t))     
        t = 0;
    end
    
    x = zeros(3,1);
    %x = create_orbit(t, 0, 0.12, 0.02);
    %x = create_orbit(t, 0, 0.6, 0.1);
    %x = create_orbit(t, 0, 1.8, 0.3);
    %x = create_orbit(t, 0, 3.0, 0.5);
    
    %{
    x = zeros(3,1);
    if (t > 2)
        x = [0 0.5 0]';
    end
    %}
    t = t + sT;
end


function Y = create_orbit(t, eta0, eta3, d_eta1)

    %最高速度
    %d_eta1 = 0.1;

    %初期時間
    t0 = 2+5;
    %加速終了時間（等速度開始時間）
    t1 = 4+5;
    %等速度終了時間（減速開始時間）
    t2 = 8+5;
    %減速終了時間
    t3 = 10+5;


    %加速終了時の位置
    eta1 = eta0 + (d_eta1*(t1-t0)/2);
    %等速終了時の位置
    eta2 = eta1 + (d_eta1*(t2-t1));

    ETA1 = [eta0 0 0 eta1 d_eta1 0]';
    ETA3 = [eta2 d_eta1 0 eta3 0 0]';

    H = [t0^5 t0^4 t0^3 t0^2 t0 1;
        5*t0^4 4*t0^3 3*t0^2 2*t0 1 0;
        20*t0^3 12*t0^2 6*t0 2 0 0;
        t1^5 t1^4 t1^3 t1^2 t1 1;
        5*t1^4 4*t1^3 3*t1^2 2*t1 1 0;
        20*t1^3 12*t1^2 6*t1 2 0 0];
    A = H\ETA1;

    H = [t2^5 t2^4 t2^3 t2^2 t2 1;
        5*t2^4 4*t2^3 3*t2^2 2*t2 1 0;
        20*t2^3 12*t2^2 6*t2 2 0 0;
        t3^5 t3^4 t3^3 t3^2 t3 1;
        5*t3^4 4*t3^3 3*t3^2 2*t3 1 0;
        20*t3^3 12*t3^2 6*t3 2 0 0];
    B = H\ETA3;


    Y = zeros(3,1);
    if (t < t0) 
        Y(1) = eta0;
        Y(2) = 0;
        Y(3) = 0;
    %加速
    elseif (t0 <= t && t < t1) 
        Y(1) = A(1)*t^5 + A(2)*t^4 + A(3)*t^3 + A(4)*t^2 + A(5)*t + A(6);
        Y(2) = 5*A(1)*t^4 + 4*A(2)*t^3 + 3*A(3)*t^2 + 2*A(4)*t + A(5);
        Y(3) = 20*A(1)*t^3 + 12*A(2)*t^2 + 6*A(3)*t + 2*A(4);
    %等速
    elseif (t1 <= t && t <= t2)
        Y(1) = (t-t1)*d_eta1 + eta1;
        Y(2) = d_eta1;
        Y(3) = 0;
    %減速
    elseif (t2 < t && t <= t3)
        Y(1) = B(1)*t^5 + B(2)*t^4 + B(3)*t^3 + B(4)*t^2 + B(5)*t + B(6);
        Y(2) = 5*B(1)*t^4 + 4*B(2)*t^3 + 3*B(3)*t^2 + 2*B(4)*t + B(5);
        Y(3) = 20*B(1)*t^3 + 12*B(2)*t^2 + 6*B(3)*t + 2*B(4);
    else
        Y(1) = eta3;
        Y(2) = 0;
        Y(3) = 0;
    end


end

== matlab function nomal_regulator/zmp/MATLAB Function1 ==
  settings: updateMethod=DISCRETE
  data: t input; u input; px output; py output; rx input; lx input
function [px,py] = fcn(t,u,rx,lx)
    
    r = -0.04;
    l = 0.04;
    xs = 0.07/2;
    ys = 0.045/2;
    
    
    r1x = (rx+xs)*u(1);
    r2x = (rx+xs)*u(2);
    r3x = (rx-xs)*u(3);
    r4x = (rx-xs)*u(4);
    PrxfRz = r1x+r2x+r3x+r4x;
    
    r1y = (r+ys)*u(1);
    r2y = (r-ys)*u(2);
    r3y = (r+ys)*u(3);
    r4y = (r-ys)*u(4);
    PryfRz = r1y+r2y+r3y+r4y;
    
    l1x = (lx+xs)*u(5);
    l2x = (lx+xs)*u(6);
    l3x = (lx-xs)*u(7);
    l4x = (lx-xs)*u(8);
    PlxfLz = l1x+l2x+l3x+l4x;
    
    l1y = (l+ys)*u(5);
    l2y = (l-ys)*u(6);
    l3y = (l+ys)*u(7);
    l4y = (l-ys)*u(8);
    PlyfLz = l1y+l2y+l3y+l4y;
    
    fRz = u(1)+u(2)+u(3)+u(4);
    fLz = u(5)+u(6)+u(7)+u(8);
    
    %両足が浮いてない
    if (fRz+fLz ~= 0 && t > 5) 
        %x軸のずれ0.02加算
        px = (PrxfRz+PlxfLz)/(fRz+fLz)+0.003;
        py = (PryfRz+PlyfLz)/(fRz+fLz)+0.005;
    else
        px = 0;
        py = 0;
    end
    
    %{
    FnR_FrontLeft
    FnR_FrontRight
    FnR_RearLeft
    FnR_RearRight
    
    
    FnL_FrontLeft
    FnL_FrontRight
    FnL_RearLeft
    FnL_RearRight
    %}
    
    
end
